simulink model "filters"  (R2017a)
settings: Solver=VariableStepAuto  StartTime=0.0  StopTime=.2736  RelTol=1e-3
InitFcn:
  | wl = 100*2*pi;
  | t=.00015;
libraries: dspfdesign x4
settings Model: Creator=frede  LastModifiedBy=frede

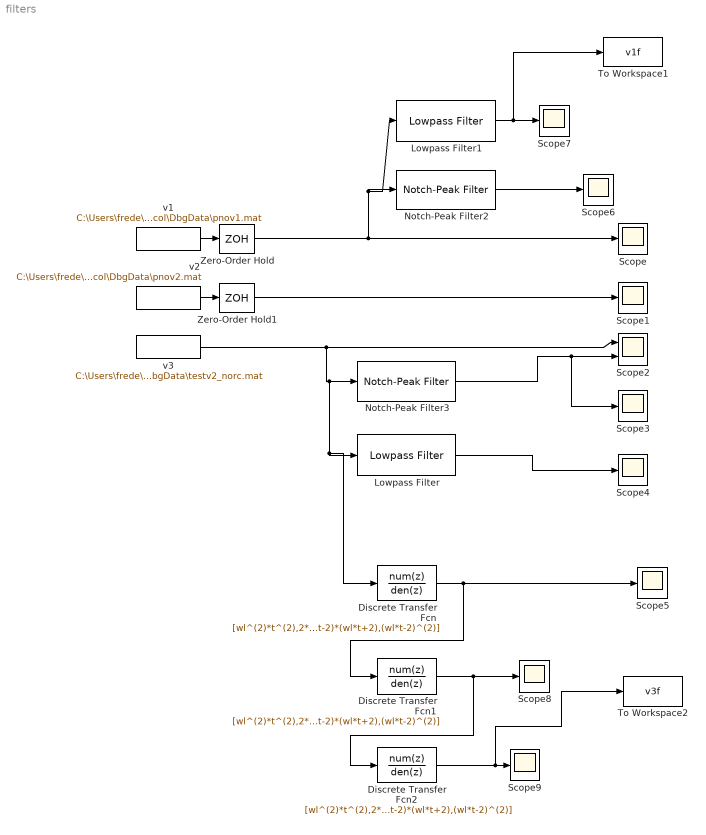
== system filters ==
  Discrete Transfer Fcn : DiscreteTransferFcn  Numerator=[wl^(2)*t^(2),2*wl^(2)*t^(2),wl^(2)*t^(2)]  Denominator=[(wl*t+2)^(2),2*(wl*t-2)*(wl*t+2),(wl*t-2)^(2)]
  Discrete Transfer Fcn1 : DiscreteTransferFcn  Numerator=[wl^(2)*t^(2),2*wl^(2)*t^(2),wl^(2)*t^(2)]  Denominator=[(wl*t+2)^(2),2*(wl*t-2)*(wl*t+2),(wl*t-2)^(2)]
  Discrete Transfer Fcn2 : DiscreteTransferFcn  Numerator=[wl^(2)*t^(2),2*wl^(2)*t^(2),wl^(2)*t^(2)]  Denominator=[(wl*t+2)^(2),2*(wl*t-2)*(wl*t+2),(wl*t-2)^(2)]
  Lowpass Filter : dspfdesign/Lowpass Filter  FilterType=FIR  DesignForMinimumOrder=on  FilterOrder=50  PassbandFrequency=100  StopbandFrequency=200  PassbandRipple=0.1  StopbandAttenuation=80  InheritSampleRate=on  SampleRate=1/.00015  SimulateUsing=Code generation  roundingMode=Floor  coeffsDataTypeStr=fixdt(1,16)
  Lowpass Filter1 : dspfdesign/Lowpass Filter  FilterType=FIR  DesignForMinimumOrder=on  FilterOrder=50  PassbandFrequency=100  StopbandFrequency=200  PassbandRipple=0.1  StopbandAttenuation=80  InheritSampleRate=on  SampleRate=1/.00015  SimulateUsing=Interpreted execution  roundingMode=Floor  coeffsDataTypeStr=fixdt(1,16)
  Notch-Peak Filter2 : dspfdesign/Notch-Peak Filter  Specification=Quality factor and center frequency  Bandwidth=200  QualityFactor=.1  CenterFrequency=1526  BandwidthCoefficient=0.72654  CenterFrequencyCoefficient=0  Output=Notch  InheritSampleRate=off  SampleRate=1/.00015  SimulateUsing=Code generation
      settings: SourceProductName=DSP System Toolbox  SourceProductBaseCode=DS
  Notch-Peak Filter3 : dspfdesign/Notch-Peak Filter  Specification=Quality factor and center frequency  Bandwidth=200  QualityFactor=.1  CenterFrequency=1526  BandwidthCoefficient=0.72654  CenterFrequencyCoefficient=0  Output=Notch  InheritSampleRate=off  SampleRate=1/.00015  SimulateUsing=Code generation
      settings: SourceProductName=DSP System Toolbox  SourceProductBaseCode=DS
  Scope{,1,3..9} (9 alike) : Scope
  Scope2 : Scope  NumInputPorts=2
  To Workspace1 : ToWorkspace  VariableName=v1f  SaveFormat=Timeseries  SampleTime=-1
  To Workspace2 : ToWorkspace  VariableName=v3f  SaveFormat=Timeseries  SampleTime=-1
  Zero-Order Hold : ZeroOrderHold  SampleTime=-1
  Zero-Order Hold1 : ZeroOrderHold  SampleTime=-1
  v1 : FromFile  FileName=C:\Users\frede\Documents\GitHub\PsoMultipleUnits\MATLAB\Protocol\DbgData\pnov1.mat  SampleTime=.00015
  v2 : FromFile  FileName=C:\Users\frede\Documents\GitHub\PsoMultipleUnits\MATLAB\Protocol\DbgData\pnov2.mat  SampleTime=.00015
  v3 : FromFile  FileName=C:\Users\frede\Documents\GitHub\PsoMultipleUnits\MATLAB\Protocol\DbgData\testv2_norc.mat  SampleTime=.00015
  wires:
  v1/1 -> Zero-Order Hold/1
  v2/1 -> Zero-Order Hold1/1
  Zero-Order Hold/1 -> Lowpass Filter1/1, Notch-Peak Filter2/1, Scope/1
  Zero-Order Hold1/1 -> Scope1/1
  v3/1 -> Notch-Peak Filter3/1, Discrete Transfer Fcn/1, Lowpass Filter/1, Scope2/1
  Notch-Peak Filter3/1 -> Scope3/1, Scope2/2
  Lowpass Filter/1 -> Scope4/1
  Discrete Transfer Fcn/1 -> Discrete Transfer Fcn1/1, Scope5/1
  Notch-Peak Filter2/1 -> Scope6/1
  Lowpass Filter1/1 -> To Workspace1/1, Scope7/1
  Discrete Transfer Fcn1/1 -> Discrete Transfer Fcn2/1, Scope8/1
  Discrete Transfer Fcn2/1 -> To Workspace2/1, Scope9/1
